simulink model "modelTest"  (R2025a)
settings: Solver=VariableStepAuto  StartTime=0.0  StopTime=10.0  MaxStep=0.0001  RelTol=1e-3
undefined symbols (not defined in the file): robot, world
libraries: simulink x1
settings Model: Creator=yaremadzulynsky  LastModifiedBy=yaremadzulynsky

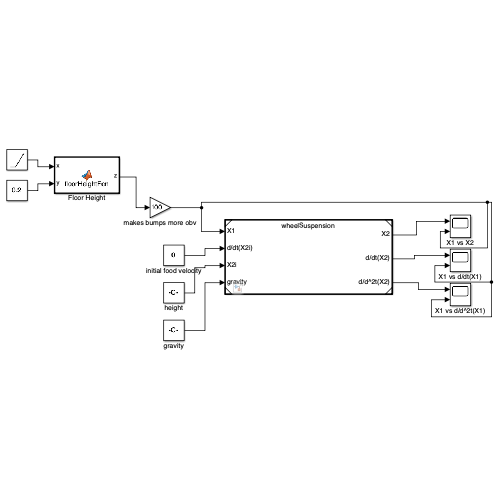
[thumbnail: Simulink's stored preview of the top-level diagram]
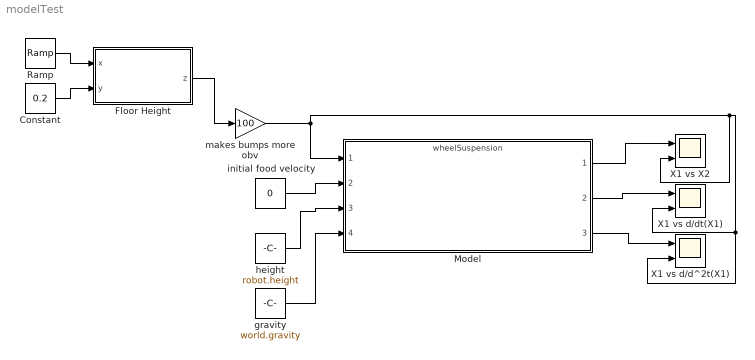
== system modelTest ==
  Constant : Constant  Value=0.2
  Floor Height : MATLAB Function  TreatAsAtomicUnit=on
  Model : ModelReference  ModelNameDialog=wheelSuspension.slx  SimulationMode=Normal  ModelReferenceVersion=1.28
  Ramp : simulink/Sources/Ramp  slope=-1  start=0  InitialOutput=0
  X1 vs X2 : Scope  NumInputPorts=2
      settings: ActiveDisplayYMinimum=4.5571520285461871  ActiveDisplayYMaximum=5.0205811298797247
  X1 vs d/d^2t(X1) : Scope  NumInputPorts=2
      settings: ActiveDisplayYMinimum=-1.2147617693969959  ActiveDisplayYMaximum=2.1836137872966082  DataLoggingVariableName=ScopeData2
  X1 vs d/dt(X1) : Scope  NumInputPorts=2
      settings: ActiveDisplayYMinimum=-0.755362167014505  ActiveDisplayYMaximum=0.55220064527891433
  gravity : Constant  Value=world.gravity
  height : Constant  Value=robot.height
  initial food velocity : Constant  Value=0
  makes bumps more obv : Gain  Gain=100
  wires:
  Model/1 -> X1 vs X2/1
  Floor Height/1(z) -> makes bumps more obv/1
  height/1 -> Model/3
  Model/3 -> X1 vs d/d^2t(X1)/1
  Model/2 -> X1 vs d/dt(X1)/1
  gravity/1 -> Model/4
  initial food velocity/1 -> Model/2
  Constant/1 -> Floor Height/2(y)
  Ramp/1 -> Floor Height/1(x)
  makes bumps more obv/1 -> Model/1, X1 vs X2/2, X1 vs d/dt(X1)/2, X1 vs d/d^2t(X1)/2

== matlab function modelTest/Floor Height ==
  data: x input; z output; y input
function z = floorHeightFcn(x, y)
%#codegen
% FLOORHEIGHTFCN  Return floor height [m] at position (x,y).
% Suitable for MATLAB Function blocks (no dynamic sizing / cat / zeros).

%% ---- CONSTANTS --------------------------------------------------------
tile_pitch          = 0.3048;  % 1 ft in m
grout_width         = 0.010;   % 1 cm in m 
grout_depth         = 0.005;   % 5 mm in m
tile_surface_height = 0.0;     % set tile height to be our datum

threshold_start_x   = -1.0;    % x coordinate of door bump
threshold_length_x  = 0.05;    % bump length 5 cm in m
threshold_height    = 0.03;    % bump height 3 cm in m
threshold_y_min     = -0.5;    % doorway span in y
threshold_y_max     =  0.5;
%% -----------------------------------------------------------------------

%% ---- TILE + GROUT -----------------------------------------------------
% local coordinates inside a tile
x_mod = x - floor(x / tile_pitch) * tile_pitch;
y_mod = y - floor(y / tile_pitch) * tile_pitch;

% distance to nearest grout line in each axis
x_dist = min(x_mod, tile_pitch - x_mod);
y_dist = min(y_mod, tile_pitch - y_mod);

% haversine–shaped grout dips
gDipX = 0.0;
if x_dist < grout_width/2
    gDipX = grout_depth/2 * (1 + cos(2*pi*x_dist/grout_width));
end

gDipY = 0.0;
if y_dist < grout_width/2
    gDipY = grout_depth/2 * (1 + cos(2*pi*y_dist/grout_width));
end

grout_valley = max(gDipX, gDipY);          % cross‑shaped groove
z_tiles      = tile_surface_height - grout_valley;   % dips negative

%% ---- DOOR THRESHOLD bump ----------------------------------------------
if  threshold_height > 0    && ...
    x >= threshold_start_x  && x <= threshold_start_x + threshold_length_x && ...
    y >= threshold_y_min    && y <= threshold_y_max

    s_local = x - threshold_start_x;       % 0 → L
    z_bump  = threshold_height/2 * ...
              (1 - cos(2*pi*s_local/threshold_length_x));   % full‑cycle haversine
    z = tile_surface_height + z_bump;      % bump sits on flat tile
else
    z = z_tiles;                           % normal tile + grout
end
end
